simulink model "Lab5_mod1"  (R2021b)
settings: Solver=ode4  StartTime=0.0  StopTime=100.0  FixedStep=2^-6  RelTol=1e-3
settings Model: Creator=JaSzw  LastModifiedBy=JaSzw

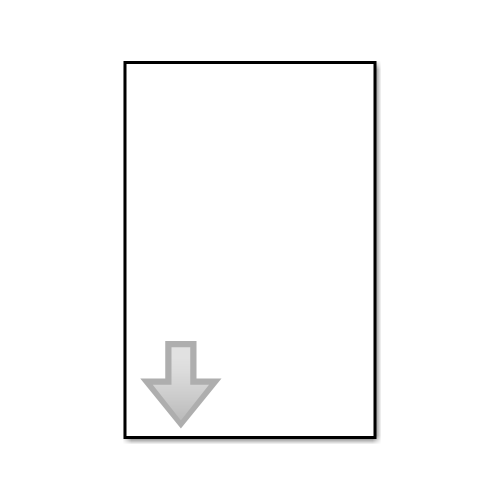
[thumbnail: Simulink's stored preview of the top-level diagram]
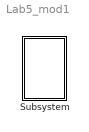
== system Lab5_mod1 ==
  Subsystem : Subsystem  mask{g=9.81, l=2, m=3, k=5, t1=12, t0=6}

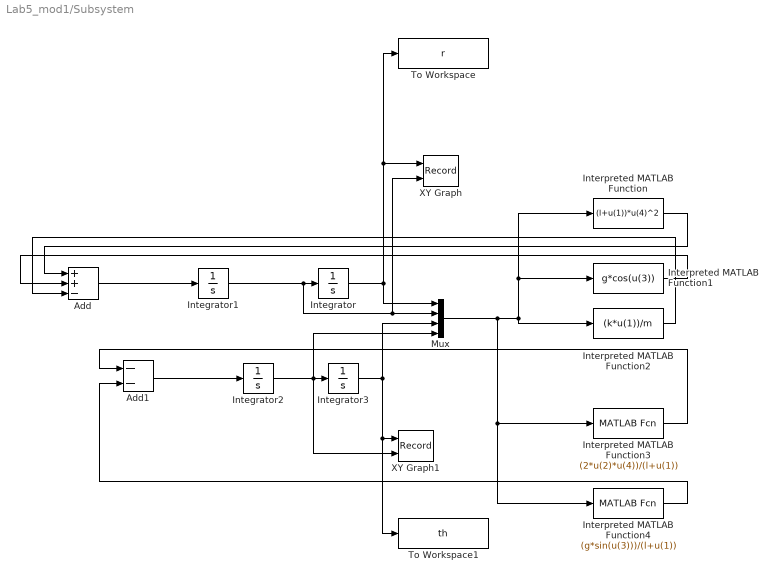
== system Lab5_mod1/Subsystem ==
  Add : Sum  Inputs=++-
  Add1 : Sum  Inputs=--
  Integrator : Integrator  InitialCondition=3
  Integrator1 : Integrator  InitialCondition=1
  Integrator2 : Integrator  InitialCondition=t1*pi/180
  Integrator3 : Integrator  InitialCondition=t0*pi/180
  Interpreted MATLAB Function : MATLABFcn  MATLABFcn=(l+u(1))*u(4)^2
  Interpreted MATLAB Function1 : MATLABFcn  MATLABFcn=g*cos(u(3))
  Interpreted MATLAB Function2 : MATLABFcn  MATLABFcn=(k*u(1))/m
  Interpreted MATLAB Function3 : MATLABFcn  MATLABFcn=(2*u(2)*u(4))/(l+u(1))
  Interpreted MATLAB Function4 : MATLABFcn  MATLABFcn=(g*sin(u(3)))/(l+u(1))
  Mux : Mux
  To Workspace : ToWorkspace  VariableName=r  SampleTime=-1
  To Workspace1 : ToWorkspace  VariableName=th  SampleTime=-1
  XY Graph : Record  FileSettingsInternal="{\"entries\":[{\"content\":{\"excelSettings\":{\"content\":{},\"type\":\"Streamout.ExcelSettings\"}},\"type\":\"Streamout.FileSettingStorage\",\"uuid\":\"e4ccd791-952d-4e57-9a9b-511e90226de0\"}],\"packageUris\":[\"http://schema.mathworks.com/mf0/streamout_blocks/R2020a\"],\"version\":\"1.0\"}"  Layout=[1 1]  SignalsInternal="{\"entries\":[{\"content\":{\"signals\":[]},\"type\":\"RecordBlkView.InputSignals\",\"uuid\":\"e7087a06-fa5a-4fb7-9820-53953387936d\"}],\"packageUris\":[\"http://schema.mathworks.com/mf0/streamout_blocks/R2020a\"],\"version\":\"1.0\"}"  VisualizationBindings="{\"xyplotplugin\":{\"info\":[{\"series\":[],\"subplotID\":1}]}}"  CompatibilityTag=XY
  XY Graph1 : Record  FileSettingsInternal="{\"entries\":[{\"content\":{\"excelSettings\":{\"content\":{},\"type\":\"Streamout.ExcelSettings\"}},\"type\":\"Streamout.FileSettingStorage\",\"uuid\":\"d7827424-ec60-4f3e-b9c9-ea8efa145648\"}],\"packageUris\":[\"http://schema.mathworks.com/mf0/streamout_blocks/R2020a\"],\"version\":\"1.0\"}"  Layout=[1 1]  SignalsInternal="{\"entries\":[{\"content\":{\"signals\":[]},\"type\":\"RecordBlkView.InputSignals\",\"uuid\":\"f7f235ff-ce1d-424c-b56a-ec2c329e3a00\"}],\"packageUris\":[\"http://schema.mathworks.com/mf0/streamout_blocks/R2020a\"],\"version\":\"1.0\"}"  VisualizationBindings="{\"xyplotplugin\":{\"info\":[{\"series\":[],\"subplotID\":1}]}}"  CompatibilityTag=XY
  wires:
  Integrator/1 -> To Workspace/1, XY Graph/1, Mux/1
  Integrator1/1 -> XY Graph/2, Mux/2, Integrator/1
  Mux/1 -> Interpreted MATLAB Function3/1, Interpreted MATLAB Function4/1, Interpreted MATLAB Function2/1, Interpreted MATLAB Function1/1, Interpreted MATLAB Function/1
  Add/1 -> Integrator1/1
  Interpreted MATLAB Function2/1 -> Add/3
  Integrator3/1 -> To Workspace1/1, XY Graph1/1, Mux/3
  Interpreted MATLAB Function4/1 -> Add1/2
  Interpreted MATLAB Function/1 -> Add/1
  Interpreted MATLAB Function1/1 -> Add/2
  Integrator2/1 -> Mux/4, XY Graph1/2, Integrator3/1
  Interpreted MATLAB Function3/1 -> Add1/1
  Add1/1 -> Integrator2/1
